simulink library "INP_EMFL"  (R2022a)
settings: Solver=VariableStepAuto  StartTime=0.0  StopTime=10.0  RelTol=1e-3
settings Model: Creator=blatak  LastModifiedBy=blatak

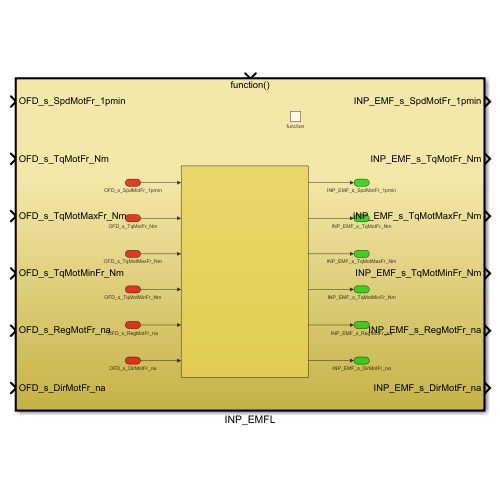
[thumbnail: Simulink's stored preview of the top-level diagram]
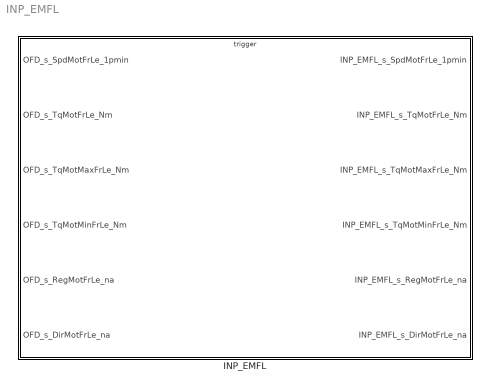
== system INP_EMFL ==
  INP_EMFL : Subsystem  TreatAsAtomicUnit=on

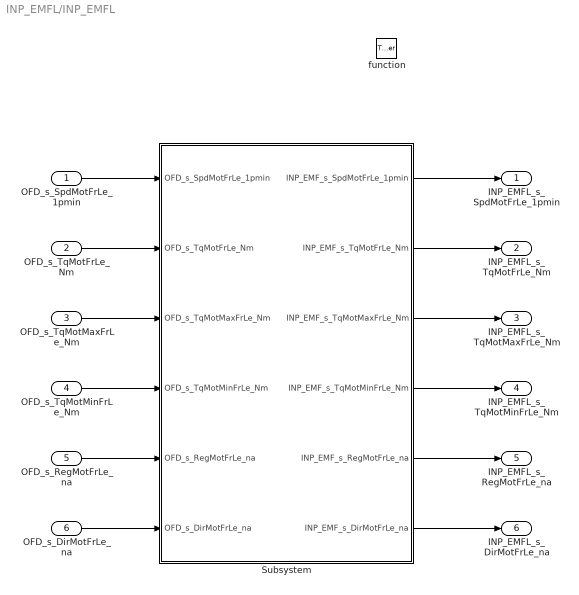
== system INP_EMFL/INP_EMFL ==
  OFD_s_SpdMotFrLe_1pmin : Inport
  OFD_s_TqMotFrLe_Nm : Inport  Port=2
  OFD_s_TqMotMaxFrLe_Nm : Inport  Port=3
  OFD_s_TqMotMinFrLe_Nm : Inport  Port=4
  OFD_s_RegMotFrLe_na : Inport  Port=5
  OFD_s_DirMotFrLe_na : Inport  Port=6
  function : TriggerPort  TriggerType=function-call  VariantControl=(inherit)
  Subsystem : Subsystem
  INP_EMFL_s_SpdMotFrLe_1pmin : Outport
  INP_EMFL_s_TqMotFrLe_Nm : Outport  Port=2
  INP_EMFL_s_TqMotMaxFrLe_Nm : Outport  Port=3
  INP_EMFL_s_TqMotMinFrLe_Nm : Outport  Port=4
  INP_EMFL_s_RegMotFrLe_na : Outport  Port=5
  INP_EMFL_s_DirMotFrLe_na : Outport  Port=6
  wires:
  OFD_s_TqMotFrLe_Nm/1 -> Subsystem/2(OFD_s_TqMotFrLe_Nm)
  OFD_s_SpdMotFrLe_1pmin/1 -> Subsystem/1(OFD_s_SpdMotFrLe_1pmin)
  Subsystem/1(INP_EMF_s_SpdMotFrLe_1pmin) -> INP_EMFL_s_SpdMotFrLe_1pmin/1
  Subsystem/2(INP_EMF_s_TqMotFrLe_Nm) -> INP_EMFL_s_TqMotFrLe_Nm/1
  OFD_s_TqMotMaxFrLe_Nm/1 -> Subsystem/3(OFD_s_TqMotMaxFrLe_Nm)
  OFD_s_TqMotMinFrLe_Nm/1 -> Subsystem/4(OFD_s_TqMotMinFrLe_Nm)
  OFD_s_RegMotFrLe_na/1 -> Subsystem/5(OFD_s_RegMotFrLe_na)
  OFD_s_DirMotFrLe_na/1 -> Subsystem/6(OFD_s_DirMotFrLe_na)
  Subsystem/3(INP_EMF_s_TqMotMaxFrLe_Nm) -> INP_EMFL_s_TqMotMaxFrLe_Nm/1
  Subsystem/4(INP_EMF_s_TqMotMinFrLe_Nm) -> INP_EMFL_s_TqMotMinFrLe_Nm/1
  Subsystem/5(INP_EMF_s_RegMotFrLe_na) -> INP_EMFL_s_RegMotFrLe_na/1
  Subsystem/6(INP_EMF_s_DirMotFrLe_na) -> INP_EMFL_s_DirMotFrLe_na/1

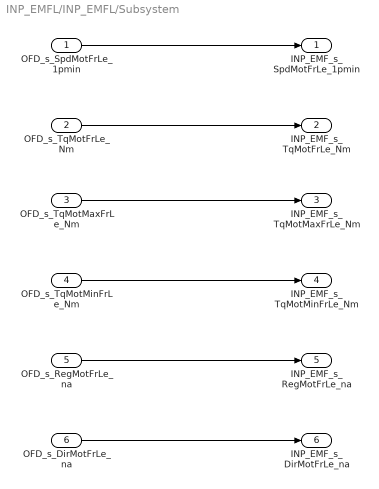
== system INP_EMFL/INP_EMFL/Subsystem ==
  OFD_s_SpdMotFrLe_1pmin : Inport
  OFD_s_TqMotFrLe_Nm : Inport  Port=2
  OFD_s_TqMotMaxFrLe_Nm : Inport  Port=3
  OFD_s_TqMotMinFrLe_Nm : Inport  Port=4
  OFD_s_RegMotFrLe_na : Inport  Port=5
  OFD_s_DirMotFrLe_na : Inport  Port=6
  INP_EMF_s_SpdMotFrLe_1pmin : Outport
  INP_EMF_s_TqMotFrLe_Nm : Outport  Port=2
  INP_EMF_s_TqMotMaxFrLe_Nm : Outport  Port=3
  INP_EMF_s_TqMotMinFrLe_Nm : Outport  Port=4
  INP_EMF_s_RegMotFrLe_na : Outport  Port=5
  INP_EMF_s_DirMotFrLe_na : Outport  Port=6
  wires:
  OFD_s_TqMotFrLe_Nm/1 -> INP_EMF_s_TqMotFrLe_Nm/1
  OFD_s_SpdMotFrLe_1pmin/1 -> INP_EMF_s_SpdMotFrLe_1pmin/1
  OFD_s_TqMotMaxFrLe_Nm/1 -> INP_EMF_s_TqMotMaxFrLe_Nm/1
  OFD_s_TqMotMinFrLe_Nm/1 -> INP_EMF_s_TqMotMinFrLe_Nm/1
  OFD_s_RegMotFrLe_na/1 -> INP_EMF_s_RegMotFrLe_na/1
  OFD_s_DirMotFrLe_na/1 -> INP_EMF_s_DirMotFrLe_na/1
